simulink model "notLinModel_S"  (R2021b)
settings: Solver=ode45  StartTime=0.0  StopTime=1  MaxStep=0.5*10^-2  RelTol=1e-9
values from neighbouring files (symbols this model uses):
  c = 0.1    [ex1.m]    (also in ex2_1.m; ex3.m; ex4.m; od.m)
  C_magnetic = 3.73e-6    (= 3.73e-06)    [ex4.m]    (also in od.m)
  gap = 3E-4    (= 0.0003)    [ex4.m]    (also in od.m)
  k = linspace(-5,5,1000)    [OP2_dynamicEstimation.m]    (also in dynamicEstimation.m = x2; ex1.m = 100; ex2_1.m = 100; ex3.m = 1272.8)
  m = 1    [ex1.m]    (also in ex2_1.m; ex3.m = 0.48; ex4.m = 0.48; od.m = 0.48)
settings Model: Creator=danli  LastModifiedBy=danli
settings SolverCC: AlgebraicLoopSolver=TrustRegion
settings DebuggingCC: SFMachineParentedDataDiag=warning

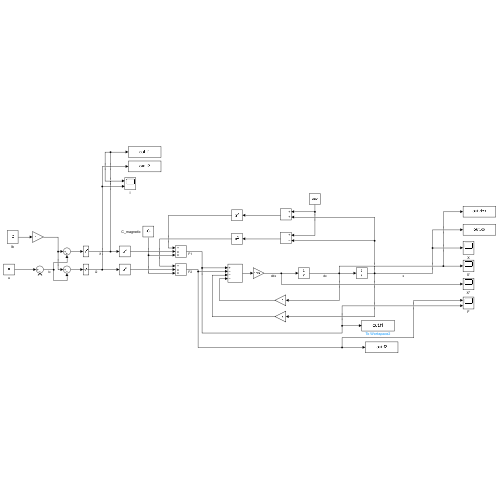
[thumbnail: Simulink's stored preview of the top-level diagram]
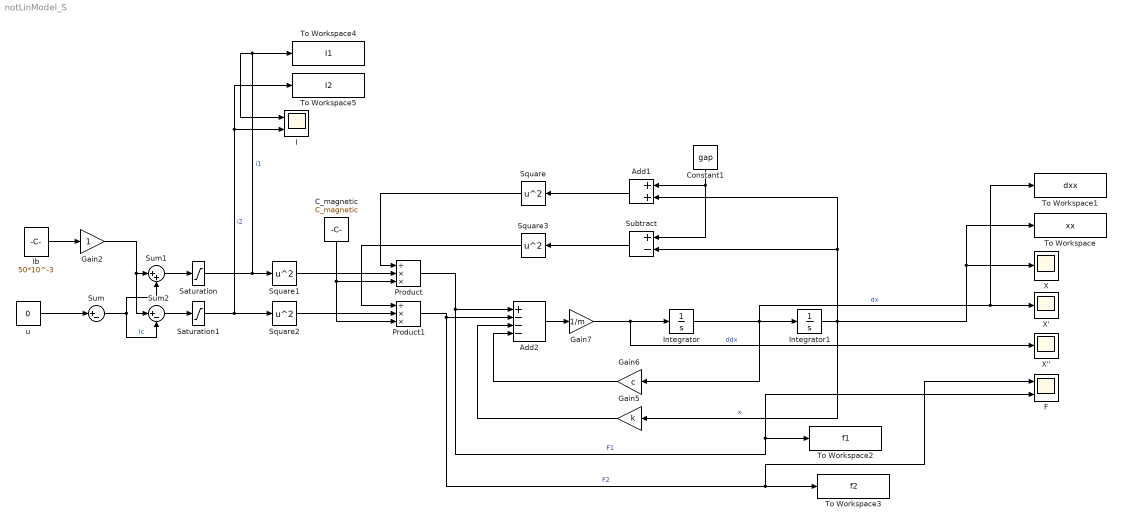
== system notLinModel_S ==
  Add1 : Sum
  Add2 : Sum  Inputs=+---
  C_magnetic : Constant  Value=C_magnetic
  Constant1 : Constant  Value=gap
  F : Scope  NumInputPorts=2
  Gain2 : Gain
  Gain5 : Gain  Gain=k
  Gain6 : Gain  Gain=c
  Gain7 : Gain  Gain=1/m
  I : Scope  NumInputPorts=2
  Ib : Constant  Value=50*10^-3
  Integrator : Integrator
  Integrator1 : Integrator  InitialCondition=50*10^-6
  Product : Product  Inputs=/**
  Product1 : Product  Inputs=/**
  Saturation : Saturate  UpperLimit=2  LowerLimit=0
  Saturation1 : Saturate  UpperLimit=2  LowerLimit=0
  Square{,1..3} (4 alike) : Math  Operator=square  SaturateOnIntegerOverflow=on
  Subtract : Sum  Inputs=+-
  Sum : Sum  Inputs=|+-
  Sum1 : Sum  Inputs=|++
  Sum2 : Sum  Inputs=|+-
  To Workspace : ToWorkspace  VariableName=xx  SaveFormat=Timeseries  SampleTime=-1
  To Workspace1 : ToWorkspace  VariableName=dxx  SaveFormat=Timeseries  SampleTime=-1
  To Workspace2 : ToWorkspace  VariableName=f1  SaveFormat=Timeseries  SampleTime=-1
  To Workspace3 : ToWorkspace  VariableName=f2  SaveFormat=Timeseries  SampleTime=-1
  To Workspace4 : ToWorkspace  VariableName=I1  SaveFormat=Timeseries  SampleTime=-1
  To Workspace5 : ToWorkspace  VariableName=I2  SaveFormat=Timeseries  SampleTime=-1
  X : Scope
  X' : Scope
  X'' : Scope
  u : Constant  Value=0
  wires:
  Ib/1 -> Gain2/1
  Sum1/1 -> Saturation/1
  Sum2/1 -> Saturation1/1
  Sum/1 -> Sum1/2, Sum2/2  "Ic"
  Gain2/1 -> Sum2/1, Sum1/1
  Integrator1/1 -> Add1/2, Subtract/2, To Workspace/1, X/1, Gain5/1  "x"
  Saturation1/1 -> I/2, To Workspace5/1, Square2/1  "i2"
  Saturation/1 -> I/1, To Workspace4/1, Square1/1  "i1"
  Square2/1 -> Product1/2
  Constant1/1 -> Subtract/1, Add1/1
  Square1/1 -> Product/2
  Gain6/1 -> Add2/4
  Integrator/1 -> Gain6/1, To Workspace1/1, X'/1, Integrator1/1  "dx"
  Gain5/1 -> Add2/3
  Product1/1 -> F/1, To Workspace3/1, Add2/2  "F2"
  Subtract/1 -> Square3/1
  Square/1 -> Product/1
  Add1/1 -> Square/1
  Add2/1 -> Gain7/1
  Product/1 -> Add2/1, F/2, To Workspace2/1  "F1"
  Square3/1 -> Product1/1
  C_magnetic/1 -> Product/3, Product1/3
  Gain7/1 -> Integrator/1, X''/1  "ddx"
  u/1 -> Sum/1
